simulink model "analyze"  (R2014a)
settings: Solver=FixedStepDiscrete  StartTime=0.0  StopTime=1  FixedStep=0.02  RelTol=1e-3
InitFcn:
  | Veh_Par_wxt
values from neighbouring files (symbols this model uses):
  ag_thr = 0.4*g    (= 3.924)    [Veh_Par_wxt.m]
  B = 2.25    [Veh_Par_wxt.m]
  bra_pre_em = 12    [Veh_Par_wxt.m]
  bra_pre_gz2 = 12/3    (= 4)    [Veh_Par_wxt.m]
  bra_pre_gz34 = 12/3    (= 4)    [Veh_Par_wxt.m]
  bra_pre_yd = 12/2    (= 6)    [Veh_Par_wxt.m]
  brakepre_dem_data = [0 1 2 3 4 5 6 7 8 9 10 11 12]    [Veh_Par_wxt.m]
  brakeTrq_dem_data = [0 218.198 436.396 654.594 872.792 1090.99 1309.188 1527.386 1745.584 1963.782 2181.98 2400.178 2618.376]    [Veh_Par_wxt.m]
  bratrq_max = 4*2618.376    (= 10473.504)    [Veh_Par_wxt.m]
  eff_tran = 0.75    [Veh_Par_wxt.m]
  G = Mass*g    (= 36297)    [Veh_Par_wxt.m]
  kd1 = 1    [Veh_Par_wxt.m]
  kd2 = 1    [Veh_Par_wxt.m]
  kd3 = 1    [Veh_Par_wxt.m]
  ki1 = 1    [Veh_Par_wxt.m]
  ki2 = 1    [Veh_Par_wxt.m]
  ki3 = 1    [Veh_Par_wxt.m]
  kp1 = 1    [Veh_Par_wxt.m]
  kp2 = 1    [Veh_Par_wxt.m]
  kp3 = 1    [Veh_Par_wxt.m]
  L = 3.12    [Veh_Par_wxt.m]
  premax = 12    [Veh_Par_wxt.m]
  Radius = 0.20    (= 0.2)    [Veh_Par_wxt.m]
  s_opt_yi_add = 0.05    [Veh_Par_wxt.m]
  s_opt_zhuan_add = 0.05    [Veh_Par_wxt.m]
  spd_map_mot = [0 100 200 300 360 400 500 600 700 800 900]*tras_ratio    [Veh_Par_wxt.m]
  spdmax = 900*tras_ratio    (= 5580)    [Veh_Par_wxt.m]
  speed_thr_park = 5/3.6/Radius*30/pi    (= 66.3145596216)    [Veh_Par_wxt.m]
  tras_ratio = 6.2    [Veh_Par_wxt.m]
  trq_map_mot = [1200 1200 1200 1200 1200 1080 864 720 617 540 480]/tras_ratio    [Veh_Par_wxt.m]
  trqmax = 80    [Veh_Par_wxt.m]
  v_thr1_b = 5    [Veh_Par_wxt.m]
  v_thr2_b = 20    [Veh_Par_wxt.m]
  v_thr_park = 5    [Veh_Par_wxt.m]
undefined symbols (not defined in the file or in its folder): DiscIntNeverNeededParam
libraries: simulink x231, ec5744lib x19
(part 13 of 16)

== system analyze/MainControl/mode_control/forward/forward/Drive/驱动防滑控制TCS ==
  trq_dem_lf : Inport
  trq_dem_lr : Inport  Port=2
  trq_dem_rf : Inport  Port=3
  trq_dem_rr : Inport  Port=4
  bra_pre_l : Inport  Port=5
  bra_pre_r : Inport  Port=6
  speed_act_lf : Inport  Port=7
  speed_act_lr : Inport  Port=8
  speed_act_rf : Inport  Port=9
  speed_act_rr : Inport  Port=10
  v_act : Inport  Port=11
  steer_dem : Inport  Port=12
  acc_y : Inport  Port=13
  brake_dem : Inport  Port=14
  s_opt_zhuan : Inport  Port=15
  MATLAB Function : MATLAB Function  TreatAsAtomicUnit=on
  Multiport Switch : MultiPortSwitch  DataPortOrder=Zero-based contiguous  Inputs=2
  Switch Case : SwitchCase  CaseConditions={0,1}  ShowDefaultCase=off
  直行TCS : Subsystem  TreatAsAtomicUnit=on
  转向TCS : Subsystem  TreatAsAtomicUnit=on
  forward_dem : Outport
  wires:
  steer_dem/1 -> 转向TCS/1(steer_dem), 直行TCS/1(steer_dem), MATLAB Function/1(steer_dem)
  MATLAB Function/1(y) -> Multiport Switch/1, Switch Case/1
  Switch Case/1 -> 转向TCS/Action
  Switch Case/2 -> 直行TCS/Action
  trq_dem_lf/1 -> 直行TCS/2(trq_dem_lf), 转向TCS/2(trq_dem_lf)
  trq_dem_lr/1 -> 直行TCS/3(trq_dem_lr), 转向TCS/3(trq_dem_lr)
  trq_dem_rf/1 -> 直行TCS/4(trq_dem_rf), 转向TCS/4(trq_dem_rf)
  trq_dem_rr/1 -> 直行TCS/5(trq_dem_rr), 转向TCS/5(trq_dem_rr)
  bra_pre_l/1 -> 直行TCS/6(bra_pre_l), 转向TCS/6(bra_pre_l)
  bra_pre_r/1 -> 直行TCS/7(bra_pre_r), 转向TCS/7(bra_pre_r)
  speed_act_lf/1 -> 直行TCS/8(speed_act_lf), 转向TCS/8(speed_act_lf)
  speed_act_lr/1 -> 直行TCS/9(speed_act_lr), 转向TCS/9(speed_act_lr)
  speed_act_rf/1 -> 直行TCS/10(speed_act_rf), 转向TCS/10(speed_act_rf)
  speed_act_rr/1 -> 直行TCS/11(speed_act_rr), 转向TCS/11(speed_act_rr)
  v_act/1 -> 直行TCS/12(v_act), 转向TCS/12(v_act)
  acc_y/1 -> 直行TCS/13(acc_y), 转向TCS/13(acc_y)
  s_opt_zhuan/1 -> 直行TCS/15(s_opt_zhuan), 转向TCS/15(s_opt_zhuan)
  brake_dem/1 -> 直行TCS/14(brake_dem), 转向TCS/14(brake_dem)
  直行TCS/1(forward_dem) -> Multiport Switch/3
  转向TCS/1(forward_dem) -> Multiport Switch/2
  Multiport Switch/1 -> forward_dem/1

== matlab function analyze/MainControl/mode_control/emergency_stop/emergency_stop/HeartBeat ==
  data: life_pre input; life output
function life = fcn(life_pre)
%#codegen
life=life_pre+1;
if life>15
    life=0;
end
end

== matlab function analyze/MainControl/mode_control/forward/forward/Drive/驱动防滑控制TCS/直行TCS/直行/MATLAB Function4 ==
  data: trq_dem_lf input; trq_dem_lr input; trq_dem_rf input; trq_dem_rr input; bra_pre_l input; bra_pre_r input; brakepre_dem input; flag_lf input; flag_lr input; trq_out_lf output; flag_rf input; flag_rr input; trq_out_lr output; trq_out_rf output; trq_out_rr output; trq_pid_lf input; trq_pid_lr input; trq_pid_rf input; trq_pid_rr input; brapre_out_l output; brapre_out_r output; mode output
function [trq_out_lf,trq_out_lr,trq_out_rf,trq_out_rr,brapre_out_l,brapre_out_r,mode] = fcn(trq_dem_lf,trq_dem_lr,trq_dem_rf,trq_dem_rr,bra_pre_l,bra_pre_r,brakepre_dem,flag_lf,flag_lr,flag_rf,flag_rr,trq_pid_lf,trq_pid_lr,trq_pid_rf,trq_pid_rr)
%#codegen pid模块在外面做，里面进行十六种情况的判断，先看一下效果，不能再修改。
if flag_lf==0 && flag_lr==0 && flag_rf==0 && flag_rr==0 % 0电机滑转===============================================0电机滑转
    trq_out_lf=trq_dem_lf;
    trq_out_lr=trq_dem_lr;
    trq_out_rf=trq_dem_rf;
    trq_out_rr=trq_dem_rr;
    brapre_out_l=bra_pre_l+brakepre_dem;
    brapre_out_r=bra_pre_r+brakepre_dem;
    mode=1;
elseif flag_lf==1 && flag_lr==0 &&flag_rf==0 && flag_rr==0 %左前轮滑转===================================================1电机滑转
    trq_out_lf=trq_pid_lf;
    trq_out_lr=trq_dem_lr+(trq_dem_lf-trq_out_lf);
    trq_out_rf=trq_dem_rf;
    trq_out_rr=trq_dem_rr;
    brapre_out_l=bra_pre_l+brakepre_dem;
    brapre_out_r=bra_pre_r+brakepre_dem;
    mode=2;
elseif flag_lf==0 && flag_lr==1 &&flag_rf==0 && flag_rr==0 %左后轮滑转
    trq_out_lr=trq_pid_lr;
    trq_out_lf=trq_dem_lf+(trq_dem_lr-trq_out_lr);
    trq_out_rf=trq_dem_rf;
    trq_out_rr=trq_dem_rr;
    brapre_out_l=bra_pre_l+brakepre_dem;
    brapre_out_r=bra_pre_r+brakepre_dem;
    mode=3;
elseif flag_lf==0 && flag_lr==0 &&flag_rf==1 && flag_rr==0 %右前轮滑转
    trq_out_rf=trq_pid_rf;
    trq_out_rr=trq_dem_rr+(trq_dem_rf-trq_out_rf);
    trq_out_lf=trq_dem_lf;
    trq_out_lr=trq_dem_lr;
    brapre_out_l=bra_pre_l+brakepre_dem;
    brapre_out_r=bra_pre_r+brakepre_dem;
    mode=4;
elseif flag_lf==0 && flag_lr==0 &&flag_rf==0 && flag_rr==1 %右后轮滑转
    trq_out_rr=trq_pid_rr;
    trq_out_rf=trq_dem_rf+(trq_dem_rr-trq_out_rr);
    trq_out_lf=trq_dem_lf;
    trq_out_lr=trq_dem_lr;
    brapre_out_l=bra_pre_l+brakepre_dem;
    brapre_out_r=bra_pre_r+brakepre_dem;
    mode=5;
elseif flag_lf==1 && flag_lr==1 &&flag_rf==0 && flag_rr==0 %左侧两轮滑转=====================================================================2电机滑转
    trq_out_lf=trq_pid_lf;
    trq_out_lr=trq_pid_lr;
    trq_out_rf=trq_dem_rf-(trq_dem_lf+trq_dem_lr-trq_out_lf-trq_out_lr)/2;
    trq_out_rr=trq_dem_rr-(trq_dem_lf+trq_dem_lr-trq_out_lf-trq_out_lr)/2;
    brapre_out_l=bra_pre_l+brakepre_dem;
    brapre_out_r=bra_pre_r+brakepre_dem;
    mode=6;
elseif flag_lf==0 && flag_lr==0 &&flag_rf==1 && flag_rr==1 %右侧两轮滑转
    trq_out_rf=trq_pid_rf;
    trq_out_rr=trq_pid_rr;
    trq_out_lf=trq_dem_lf-(trq_dem_rf+trq_dem_rr-trq_out_rf-trq_out_rr)/2;
    trq_out_lr=trq_dem_lr-(trq_dem_rf+trq_dem_rr-trq_out_rf-trq_out_rr)/2;
    brapre_out_l=bra_pre_l+brakepre_dem;
    brapre_out_r=bra_pre_r+brakepre_dem;
    mode=7;
elseif flag_lf==1 && flag_lr==0 &&flag_rf==1 && flag_rr==0 %前轴滑转
    trq_out_lf=trq_pid_lf;
    trq_out_lr=trq_dem_lr+(trq_dem_lf-trq_out_lf);
    trq_out_rf=trq_pid_rf;
    trq_out_rr=trq_dem_rr+(trq_dem_rf-trq_out_rf);
    brapre_out_l=bra_pre_l+brakepre_dem;
    brapre_out_r=bra_pre_r+brakepre_dem;
    mode=8;
elseif flag_lf==0 && flag_lr==1 &&flag_rf==0 && flag_rr==1 %后轴滑转
    trq_out_lr=trq_pid_lr;
    trq_out_lf=trq_dem_lf+(trq_dem_lr-trq_out_lr);
    trq_out_rr=trq_pid_rr;
    trq_out_rf=trq_dem_rf+(trq_dem_rr-trq_out_rr);
    brapre_out_l=bra_pre_l+brakepre_dem;
    brapre_out_r=bra_pre_r+brakepre_dem;
    mode=9;
elseif flag_lf==1 && flag_lr==0 &&flag_rf==0 && flag_rr==1 %左前轮和右后轮滑转
    trq_out_lf=trq_pid_lf;
    trq_out_lr=trq_dem_lr+(trq_dem_lf-trq_out_lf);
    trq_out_rr=trq_pid_rr;
    trq_out_rf=trq_dem_rf+(trq_dem_rr-trq_out_rr);
    brapre_out_l=bra_pre_l+brakepre_dem;
    brapre_out_r=bra_pre_r+brakepre_dem;
    mode=10;
elseif flag_lf==0 && flag_lr==1 &&flag_rf==1 && flag_rr==0 %左后轮和右前轮滑转
    trq_out_lr=trq_pid_lr;
    trq_out_lf=trq_dem_lf+(trq_dem_lr-trq_out_lr);
    trq_out_rf=trq_pid_rf;
    trq_out_rr=trq_dem_rr+(trq_dem_rf-trq_out_rf);
    brapre_out_l=bra_pre_l+brakepre_dem;
    brapre_out_r=bra_pre_r+brakepre_dem;
    mode=11;
elseif flag_lf==1 && flag_lr==1 &&flag_rf==1 && flag_rr==0 %右后不滑转======================================================================3电机滑转
    trq_out_lf=trq_pid_lf;
    trq_out_lr=trq_pid_lr;
    trq_out_rf=trq_pid_rf;
    trq_out_rr=trq_dem_rr+(trq_dem_rf-trq_out_rf)-(trq_dem_lf+trq_dem_lr-trq_out_lf-trq_out_lr);
    brapre_out_l=bra_pre_l+brakepre_dem;
    brapre_out_r=bra_pre_r+brakepre_dem;
    mode=12;
elseif flag_lf==1 && flag_lr==1 &&flag_rf==0 && flag_rr==1 %右前不滑转
    trq_out_lf=trq_pid_lf;
    trq_out_lr=trq_pid_lr;
    trq_out_rr=trq_pid_rr;
    trq_out_rf=trq_dem_rf+(trq_dem_rr-trq_out_rr)-(trq_dem_lf+trq_dem_lr-trq_out_lf-trq_out_lr);
    brapre_out_l=bra_pre_l+brakepre_dem;
    brapre_out_r=bra_pre_r+brakepre_dem;
    mode=13;
elseif flag_lf==1 && flag_lr==0 &&flag_rf==1 && flag_rr==1 %左后不滑转
    trq_out_rf=trq_pid_rf;
    trq_out_rr=trq_pid_rr;
    trq_out_lf=trq_pid_lf;
    trq_out_lr=trq_dem_lr+(trq_dem_lf-trq_out_lf)-(trq_dem_rf+trq_dem_rr-trq_out_rf-trq_out_rr);
    brapre_out_l=bra_pre_l+brakepre_dem;
    brapre_out_r=bra_pre_r+brakepre_dem;
    mode=14;
elseif flag_lf==0 && flag_lr==1 &&flag_rf==1 && flag_rr==1 %左前不滑转
    trq_out_rf=trq_pid_rf;
    trq_out_rr=trq_pid_rr;
    trq_out_lr=trq_pid_lr;
    trq_out_lf=trq_dem_lf+(trq_dem_lr-trq_out_lr)-(trq_dem_rf+trq_dem_rr-trq_out_rf-trq_out_rr);
    brapre_out_l=bra_pre_l+brakepre_dem;
    brapre_out_r=bra_pre_r+brakepre_dem;
    mode=15;
else
    %     flag_lf==1 && flag_lr==1 &&flag_rf==1 && flag_rr==1 %4电机均滑转======================================================================4电机均滑转
    trqcha=(trq_pid_lf+trq_pid_lr)-(trq_pid_rf+trq_pid_rr);
    if trqcha>0
        trq_out_rf=trq_pid_rf;
        trq_out_rr=trq_pid_rr;
        trq_out_lf=trq_pid_lf-(trq_pid_lf/(trq_pid_lf+trq_pid_lr))*trqcha;
        trq_out_lr=trq_pid_lr-(trq_pid_lr/(trq_pid_lf+trq_pid_lr))*trqcha;
    else
        trq_out_lf=trq_pid_lf;
        trq_out_lr=trq_pid_lr;
        trq_out_rf=trq_pid_rf+(trq_pid_rf/(trq_pid_rf+trq_pid_rr))*trqcha;
        trq_out_rr=trq_pid_rr+(trq_pid_rr/(trq_pid_rf+trq_pid_rr))*trqcha;
    end
    brapre_out_l=bra_pre_l+brakepre_dem;
    brapre_out_r=bra_pre_r+brakepre_dem;
    mode=16;
end
trq_out_lf=max(0,trq_out_lf);
trq_out_lr=max(0,trq_out_lr);
trq_out_rf=max(0,trq_out_rf);
trq_out_rr=max(0,trq_out_rr);
brapre_out_l=brapre_out_l;
brapre_out_r=brapre_out_r;
end

== system analyze/MainControl/mode_control/backward/backward/Drive/驱动防滑控制TCS/直行TCS ==
  steer_dem : Inport
  trq_dem_lf : Inport  Port=2
  trq_dem_lr : Inport  Port=3
  trq_dem_rf : Inport  Port=4
  trq_dem_rr : Inport  Port=5
  bra_pre_l : Inport  Port=6
  bra_pre_r : Inport  Port=7
  speed_act_lf : Inport  Port=8
  speed_act_lr : Inport  Port=9
  speed_act_rf : Inport  Port=10
  speed_act_rr : Inport  Port=11
  v_act : Inport  Port=12
  acc_y : Inport  Port=13
  brake_dem : Inport  Port=14
  s_opt_zhuan : Inport  Port=15
  Action Port : ActionPort  ActionType=case
  Scope : Scope  NumInputPorts=4
      settings: YMin=-5~-5~-5~-5  YMax=5~5~5~5  SaveName=ScopeData42
  Subsystem : Subsystem
  Subsystem1 : Subsystem
  Subsystem2 : Subsystem
  Subsystem3 : Subsystem
  Terminator : Terminator
  Terminator1 : Terminator
  直行 : Subsystem  TreatAsAtomicUnit=on
  backward_dem : Outport
  wires:
  steer_dem/1 -> Terminator1/1
  speed_act_lf/1 -> Subsystem/1(speed_act_lf)
  v_act/1 -> Subsystem2/2(v_act), Subsystem1/2(v_act), Subsystem/2(v_act), Subsystem3/2(v_act)
  speed_act_lr/1 -> Subsystem1/1(speed_act_lr)
  speed_act_rf/1 -> Subsystem2/1(speed_act_rf)
  speed_act_rr/1 -> Subsystem3/1(speed_act_rr)
  acc_y/1 -> Terminator/1
  trq_dem_lr/1 -> 直行/2(trq_dem_lr)
  trq_dem_lf/1 -> 直行/1(trq_dem_lf)
  trq_dem_rf/1 -> 直行/3(trq_dem_rf)
  trq_dem_rr/1 -> 直行/4(trq_dem_rr)
  bra_pre_l/1 -> 直行/5(bra_pre_l)
  bra_pre_r/1 -> 直行/6(bra_pre_r)
  Subsystem/1(s_act_lf) -> 直行/7(s_act_lf), Scope/1
  Subsystem1/1(s_act_lr) -> 直行/8(s_act_lr), Scope/2
  Subsystem2/1(s_act_rf) -> 直行/9(s_act_rf), Scope/3
  Subsystem3/1(s_act_rr) -> 直行/10(s_act_rr), Scope/4
  s_opt_zhuan/1 -> 直行/12(s_opt_zhuan)
  brake_dem/1 -> 直行/11(brake_dem)
  直行/1(backward_dem) -> backward_dem/1

== system analyze/MainControl/mode_control/backward/backward/Drive/驱动防滑控制TCS/转向TCS ==
  steer_dem : Inport
  trq_dem_lf : Inport  Port=2
  trq_dem_lr : Inport  Port=3
  trq_dem_rf : Inport  Port=4
  trq_dem_rr : Inport  Port=5
  bra_pre_l : Inport  Port=6
  bra_pre_r : Inport  Port=7
  speed_act_lf : Inport  Port=8
  speed_act_lr : Inport  Port=9
  speed_act_rf : Inport  Port=10
  speed_act_rr : Inport  Port=11
  v_act : Inport  Port=12
  acc_y : Inport  Port=13
  brake_dem : Inport  Port=14
  s_opt_zhuan : Inport  Port=15
  Action Port : ActionPort  ActionType=case
  MATLAB Function : MATLAB Function  TreatAsAtomicUnit=on
  Multiport Switch : MultiPortSwitch  DataPortOrder=Zero-based contiguous  Inputs=2
  Subsystem : Subsystem
  Subsystem1 : Subsystem
  Subsystem2 : Subsystem
  Subsystem3 : Subsystem
  Switch Case : SwitchCase  CaseConditions={0,1}  ShowDefaultCase=off
  Terminator : Terminator
  右转 : Subsystem  TreatAsAtomicUnit=on
  左转 : Subsystem  TreatAsAtomicUnit=on
  backward_dem : Outport
  wires:
  Multiport Switch/1 -> backward_dem/1
  右转/1(backward_dem) -> Multiport Switch/3
  左转/1(backward_dem) -> Multiport Switch/2
  brake_dem/1 -> 左转/11(brake_dem), 右转/11(brake_dem)
  s_opt_zhuan/1 -> 左转/12(s_opt_zhuan), 右转/12(s_opt_zhuan)
  Subsystem3/1(s_act_rr) -> 左转/10(s_act_rr), 右转/10(s_act_rr)
  Subsystem2/1(s_act_rf) -> 左转/9(s_act_rf), 右转/9(s_act_rf)
  Subsystem1/1(s_act_lr) -> 左转/8(s_act_lr), 右转/8(s_act_lr)
  Subsystem/1(s_act_lf) -> 左转/7(s_act_lf), 右转/7(s_act_lf)
  bra_pre_r/1 -> 左转/6(bra_pre_r), 右转/6(bra_pre_r)
  bra_pre_l/1 -> 左转/5(bra_pre_l), 右转/5(bra_pre_l)
  trq_dem_rr/1 -> 左转/4(trq_dem_rr), 右转/4(trq_dem_rr)
  trq_dem_rf/1 -> 左转/3(trq_dem_rf), 右转/3(trq_dem_rf)
  trq_dem_lf/1 -> 左转/1(trq_dem_lf), 右转/1(trq_dem_lf)
  trq_dem_lr/1 -> 左转/2(trq_dem_lr), 右转/2(trq_dem_lr)
  acc_y/1 -> Terminator/1
  Switch Case/2 -> 右转/Action
  Switch Case/1 -> 左转/Action
  speed_act_rr/1 -> Subsystem3/1(speed_act_rr)
  speed_act_rf/1 -> Subsystem2/1(speed_act_rf)
  speed_act_lr/1 -> Subsystem1/1(speed_act_lr)
  v_act/1 -> Subsystem3/2(v_act), Subsystem/2(v_act), Subsystem1/2(v_act), Subsystem2/2(v_act)
  speed_act_lf/1 -> Subsystem/1(speed_act_lf)
  MATLAB Function/1(y) -> Switch Case/1, Multiport Switch/1
  steer_dem/1 -> MATLAB Function/1(steer_dem)

== system analyze/MainControl/mode_control/forward/forward/Drive/驱动防滑控制TCS/直行TCS ==
  steer_dem : Inport
  trq_dem_lf : Inport  Port=2
  trq_dem_lr : Inport  Port=3
  trq_dem_rf : Inport  Port=4
  trq_dem_rr : Inport  Port=5
  bra_pre_l : Inport  Port=6
  bra_pre_r : Inport  Port=7
  speed_act_lf : Inport  Port=8
  speed_act_lr : Inport  Port=9
  speed_act_rf : Inport  Port=10
  speed_act_rr : Inport  Port=11
  v_act : Inport  Port=12
  acc_y : Inport  Port=13
  brake_dem : Inport  Port=14
  s_opt_zhuan : Inport  Port=15
  Action Port : ActionPort  ActionType=case
  Scope : Scope  NumInputPorts=4
      settings: YMin=-5~-5~-5~-5  YMax=5~5~5~5  SaveName=ScopeData42
  Subsystem : Subsystem
  Subsystem1 : Subsystem
  Subsystem2 : Subsystem
  Subsystem3 : Subsystem
  Terminator : Terminator
  Terminator1 : Terminator
  直行 : Subsystem  TreatAsAtomicUnit=on
  forward_dem : Outport
  wires:
  直行/1(forward_dem) -> forward_dem/1
  brake_dem/1 -> 直行/11(brake_dem)
  s_opt_zhuan/1 -> 直行/12(s_opt_zhuan)
  Subsystem3/1(s_act_rr) -> Scope/4, 直行/10(s_act_rr)
  Subsystem2/1(s_act_rf) -> Scope/3, 直行/9(s_act_rf)
  Subsystem1/1(s_act_lr) -> Scope/2, 直行/8(s_act_lr)
  Subsystem/1(s_act_lf) -> Scope/1, 直行/7(s_act_lf)
  bra_pre_r/1 -> 直行/6(bra_pre_r)
  bra_pre_l/1 -> 直行/5(bra_pre_l)
  trq_dem_rr/1 -> 直行/4(trq_dem_rr)
  trq_dem_rf/1 -> 直行/3(trq_dem_rf)
  trq_dem_lf/1 -> 直行/1(trq_dem_lf)
  trq_dem_lr/1 -> 直行/2(trq_dem_lr)
  acc_y/1 -> Terminator/1
  speed_act_rr/1 -> Subsystem3/1(speed_act_rr)
  speed_act_rf/1 -> Subsystem2/1(speed_act_rf)
  speed_act_lr/1 -> Subsystem1/1(speed_act_lr)
  v_act/1 -> Subsystem3/2(v_act), Subsystem/2(v_act), Subsystem1/2(v_act), Subsystem2/2(v_act)
  speed_act_lf/1 -> Subsystem/1(speed_act_lf)
  steer_dem/1 -> Terminator1/1

== system analyze/MainControl/mode_control/forward/forward/Drive/驱动防滑控制TCS/转向TCS ==
  steer_dem : Inport
  trq_dem_lf : Inport  Port=2
  trq_dem_lr : Inport  Port=3
  trq_dem_rf : Inport  Port=4
  trq_dem_rr : Inport  Port=5
  bra_pre_l : Inport  Port=6
  bra_pre_r : Inport  Port=7
  speed_act_lf : Inport  Port=8
  speed_act_lr : Inport  Port=9
  speed_act_rf : Inport  Port=10
  speed_act_rr : Inport  Port=11
  v_act : Inport  Port=12
  acc_y : Inport  Port=13
  brake_dem : Inport  Port=14
  s_opt_zhuan : Inport  Port=15
  Action Port : ActionPort  ActionType=case
  MATLAB Function : MATLAB Function  TreatAsAtomicUnit=on
  Multiport Switch : MultiPortSwitch  DataPortOrder=Zero-based contiguous  Inputs=2
  Subsystem : Subsystem
  Subsystem1 : Subsystem
  Subsystem2 : Subsystem
  Subsystem3 : Subsystem
  Switch Case : SwitchCase  CaseConditions={0,1}  ShowDefaultCase=off
  Terminator : Terminator
  右转 : Subsystem  TreatAsAtomicUnit=on
  左转 : Subsystem  TreatAsAtomicUnit=on
  forward_dem : Outport
  wires:
  steer_dem/1 -> MATLAB Function/1(steer_dem)
  MATLAB Function/1(y) -> Multiport Switch/1, Switch Case/1
  speed_act_lf/1 -> Subsystem/1(speed_act_lf)
  v_act/1 -> Subsystem2/2(v_act), Subsystem1/2(v_act), Subsystem/2(v_act), Subsystem3/2(v_act)
  speed_act_lr/1 -> Subsystem1/1(speed_act_lr)
  speed_act_rf/1 -> Subsystem2/1(speed_act_rf)
  speed_act_rr/1 -> Subsystem3/1(speed_act_rr)
  Switch Case/1 -> 左转/Action
  Switch Case/2 -> 右转/Action
  acc_y/1 -> Terminator/1
  trq_dem_lr/1 -> 右转/2(trq_dem_lr), 左转/2(trq_dem_lr)
  trq_dem_lf/1 -> 右转/1(trq_dem_lf), 左转/1(trq_dem_lf)
  trq_dem_rf/1 -> 右转/3(trq_dem_rf), 左转/3(trq_dem_rf)
  trq_dem_rr/1 -> 右转/4(trq_dem_rr), 左转/4(trq_dem_rr)
  bra_pre_l/1 -> 右转/5(bra_pre_l), 左转/5(bra_pre_l)
  bra_pre_r/1 -> 右转/6(bra_pre_r), 左转/6(bra_pre_r)
  Subsystem/1(s_act_lf) -> 右转/7(s_act_lf), 左转/7(s_act_lf)
  Subsystem1/1(s_act_lr) -> 右转/8(s_act_lr), 左转/8(s_act_lr)
  Subsystem2/1(s_act_rf) -> 右转/9(s_act_rf), 左转/9(s_act_rf)
  Subsystem3/1(s_act_rr) -> 右转/10(s_act_rr), 左转/10(s_act_rr)
  s_opt_zhuan/1 -> 右转/12(s_opt_zhuan), 左转/12(s_opt_zhuan)
  brake_dem/1 -> 右转/11(brake_dem), 左转/11(brake_dem)
  左转/1(forward_dem) -> Multiport Switch/2
  右转/1(forward_dem) -> Multiport Switch/3
  Multiport Switch/1 -> forward_dem/1

== system analyze/MainControl/mode_control/backward/backward/Drive/驱动防滑控制TCS/直行TCS/Subsystem ==
  speed_act_lf : Inport
  v_act : Inport  Port=2
  Add : Sum
  Constant : Constant  Value=eps
  Divide : Product  Inputs=*/
  Gain : Gain  Gain=pi/30
  Gain1 : Gain  Gain=Radius
  Gain2 : Gain  Gain=1/3.6
  Subtract : Sum  Inputs=+-
  s_act_lf : Outport
  wires:
  speed_act_lf/1 -> Gain/1
  Gain/1 -> Gain1/1
  v_act/1 -> Gain2/1
  Gain1/1 -> Add/1, Subtract/1
  Gain2/1 -> Subtract/2
  Subtract/1 -> Divide/1
  Constant/1 -> Add/2
  Add/1 -> Divide/2
  Divide/1 -> s_act_lf/1

== system analyze/MainControl/mode_control/backward/backward/Drive/驱动防滑控制TCS/直行TCS/Subsystem1 ==
  speed_act_lr : Inport
  v_act : Inport  Port=2
  Add : Sum
  Constant : Constant  Value=eps
  Divide : Product  Inputs=*/
  Gain : Gain  Gain=pi/30
  Gain1 : Gain  Gain=Radius
  Gain2 : Gain  Gain=1/3.6
  Subtract : Sum  Inputs=+-
  s_act_lr : Outport
  wires:
  Divide/1 -> s_act_lr/1
  Add/1 -> Divide/2
  Constant/1 -> Add/2
  Subtract/1 -> Divide/1
  Gain2/1 -> Subtract/2
  Gain1/1 -> Subtract/1, Add/1
  v_act/1 -> Gain2/1
  Gain/1 -> Gain1/1
  speed_act_lr/1 -> Gain/1

== system analyze/MainControl/mode_control/backward/backward/Drive/驱动防滑控制TCS/直行TCS/Subsystem2 ==
  speed_act_rf : Inport
  v_act : Inport  Port=2
  Add : Sum
  Constant : Constant  Value=eps
  Divide : Product  Inputs=*/
  Gain : Gain  Gain=pi/30
  Gain1 : Gain  Gain=Radius
  Gain2 : Gain  Gain=1/3.6
  Subtract : Sum  Inputs=+-
  s_act_rf : Outport
  wires:
  speed_act_rf/1 -> Gain/1
  Gain/1 -> Gain1/1
  v_act/1 -> Gain2/1
  Gain1/1 -> Add/1, Subtract/1
  Gain2/1 -> Subtract/2
  Subtract/1 -> Divide/1
  Constant/1 -> Add/2
  Add/1 -> Divide/2
  Divide/1 -> s_act_rf/1

== system analyze/MainControl/mode_control/backward/backward/Drive/驱动防滑控制TCS/直行TCS/Subsystem3 ==
  speed_act_rr : Inport
  v_act : Inport  Port=2
  Add : Sum
  Constant : Constant  Value=eps
  Divide : Product  Inputs=*/
  Gain : Gain  Gain=pi/30
  Gain1 : Gain  Gain=Radius
  Gain2 : Gain  Gain=1/3.6
  Subtract : Sum  Inputs=+-
  s_act_rr : Outport
  wires:
  Divide/1 -> s_act_rr/1
  Add/1 -> Divide/2
  Constant/1 -> Add/2
  Subtract/1 -> Divide/1
  Gain2/1 -> Subtract/2
  Gain1/1 -> Subtract/1, Add/1
  v_act/1 -> Gain2/1
  Gain/1 -> Gain1/1
  speed_act_rr/1 -> Gain/1

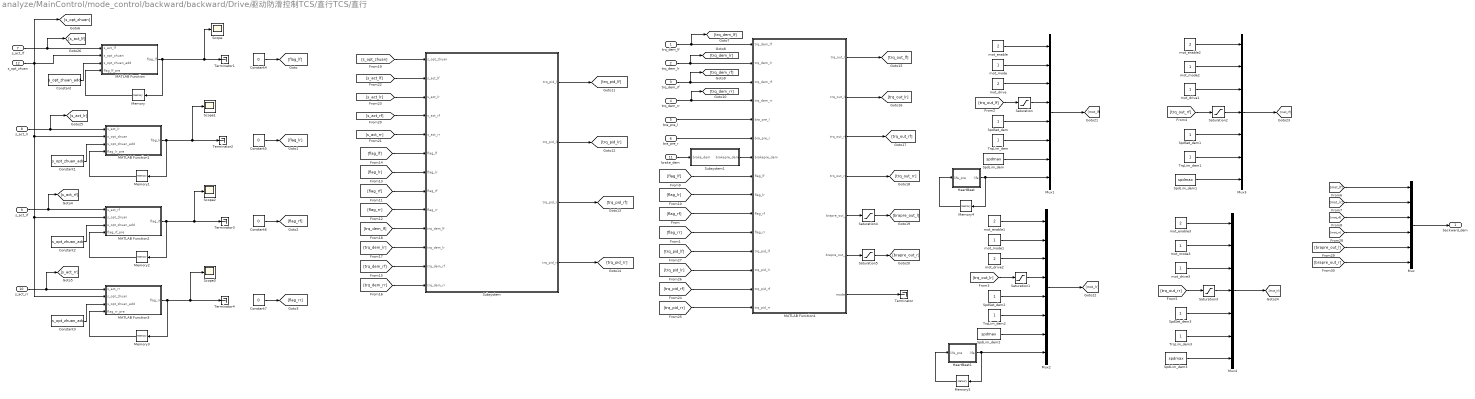
== system analyze/MainControl/mode_control/backward/backward/Drive/驱动防滑控制TCS/直行TCS/直行 ==
  trq_dem_lf : Inport
  trq_dem_lr : Inport  Port=2
  trq_dem_rf : Inport  Port=3
  trq_dem_rr : Inport  Port=4
  bra_pre_l : Inport  Port=5
  bra_pre_r : Inport  Port=6
  s_act_lf : Inport  Port=7
  s_act_lr : Inport  Port=8
  s_act_rf : Inport  Port=9
  s_act_rr : Inport  Port=10
  brake_dem : Inport  Port=11
  s_opt_zhuan : Inport  Port=12
  Constant{,1..3} (4 alike) : Constant  Value=s_opt_zhuan_add
  Constant{4..7} (4 alike) : Constant  Value=0
  HeartBeat : MATLAB Function  TreatAsAtomicUnit=on
  HeartBeat1 : MATLAB Function  TreatAsAtomicUnit=on
  MATLAB Function : MATLAB Function  TreatAsAtomicUnit=on
  MATLAB Function1 : MATLAB Function  TreatAsAtomicUnit=on
  MATLAB Function2 : MATLAB Function  TreatAsAtomicUnit=on
  MATLAB Function3 : MATLAB Function  TreatAsAtomicUnit=on
  MATLAB Function4 : MATLAB Function  TreatAsAtomicUnit=on
  Memory{,1..5} (6 alike) : Memory  InheritSampleTime=on
  Mux : Mux  Inputs=6
  Mux1 : Mux  Inputs=8
  Mux2 : Mux  Inputs=8
  Mux3 : Mux  Inputs=7
  Mux4 : Mux  Inputs=7
  Saturation{,1..3} (4 alike) : Saturate  UpperLimit=trqmax  LowerLimit=0
  Saturation4 : Saturate  UpperLimit=premax  LowerLimit=0
  Saturation5 : Saturate  UpperLimit=premax  LowerLimit=0
  Scope{,1..3} (4 alike) : Scope
      Scope settings: SaveName=ScopeData43
      Scope1 settings: SaveName=ScopeData44
      Scope2 settings: SaveName=ScopeData45
      Scope3 settings: SaveName=ScopeData46
  SpdLim_dem{,1..3} (4 alike) : Constant  Value=spdmax
  SpdSet_dem{,1..3} (4 alike) : Constant
  Subsystem : Subsystem
  Subsystem1 : Subsystem
  Terminator{,1..4} (5 alike) : Terminator
  TrqLim_dem{,1..3} (4 alike) : Constant
  mot_drive : Constant  Value=2
  mot_drive1 : Constant
  mot_drive2 : Constant  Value=2
  mot_drive3 : Constant
  mot_enable{,1..3} (4 alike) : Constant  Value=2
  mot_mode{,1..3} (4 alike) : Constant
  backward_dem : Outport
  wires:
  Saturation5/1 -> [brapre_out_r]
  Saturation4/1 -> [brapre_out_l]
  Saturation3/1 -> Mux4/4
  Saturation1/1 -> Mux2/4
  Saturation2/1 -> Mux3/4
  Saturation/1 -> Mux1/4
  MATLAB Function4/7(mode) -> Terminator/1
  brake_dem/1 -> Subsystem1/1(brake_dem)
  Subsystem1/1(brakepre_dem) -> MATLAB Function4/7(brakepre_dem)
  [brapre_out_r] -> Mux/6
  [brapre_out_l] -> Mux/5
  [mot_rr] -> Mux/4
  [mot_rf] -> Mux/3
  [mot_lr] -> Mux/2
  [mot_lf] -> Mux/1
  MATLAB Function4/6(brapre_out_r) -> Saturation5/1
  MATLAB Function4/5(brapre_out_l) -> Saturation4/1
  MATLAB Function4/4(trq_out_rr) -> [trq_out_rr]
  MATLAB Function4/3(trq_out_rf) -> [trq_out_rf]
  MATLAB Function4/2(trq_out_lr) -> [trq_out_lr]
  MATLAB Function4/1(trq_out_lf) -> [trq_out_lf]
  mot_drive/1 -> Mux1/3
  mot_mode/1 -> Mux1/2
  [trq_out_lf] -> Saturation/1
  mot_enable/1 -> Mux1/1
  SpdSet_dem/1 -> Mux1/5
  Mux1/1 -> [mot_lf]
  TrqLim_dem/1 -> Mux1/6
  HeartBeat/1(life) -> Mux1/8, Memory4/1
  Memory4/1 -> HeartBeat/1(life_pre)
  SpdLim_dem/1 -> Mux1/7
  mot_drive1/1 -> Mux3/3
  mot_mode2/1 -> Mux3/2
  [trq_out_rf] -> Saturation2/1
  mot_enable2/1 -> Mux3/1
  SpdSet_dem1/1 -> Mux3/5
  Mux3/1 -> [mot_rf]
  TrqLim_dem1/1 -> Mux3/6
  SpdLim_dem1/1 -> Mux3/7
  mot_drive2/1 -> Mux2/3
  mot_mode1/1 -> Mux2/2
  [trq_out_lr] -> Saturation1/1
  mot_enable1/1 -> Mux2/1
  SpdSet_dem2/1 -> Mux2/5
  Mux2/1 -> [mot_lr]
  TrqLim_dem2/1 -> Mux2/6
  HeartBeat1/1(life) -> Mux2/8, Memory5/1
  Memory5/1 -> HeartBeat1/1(life_pre)
  SpdLim_dem2/1 -> Mux2/7
  mot_drive3/1 -> Mux4/3
  mot_mode3/1 -> Mux4/2
  [trq_out_rr] -> Saturation3/1
  mot_enable3/1 -> Mux4/1
  SpdSet_dem3/1 -> Mux4/5
  Mux4/1 -> [mot_rr]
  TrqLim_dem3/1 -> Mux4/6
  SpdLim_dem3/1 -> Mux4/7
  bra_pre_r/1 -> MATLAB Function4/6(bra_pre_r)
  bra_pre_l/1 -> MATLAB Function4/5(bra_pre_l)
  trq_dem_rr/1 -> [trq_dem_rr], MATLAB Function4/4(trq_dem_rr)
  trq_dem_rf/1 -> [trq_dem_rf], MATLAB Function4/3(trq_dem_rf)
  trq_dem_lr/1 -> [trq_dem_lr], MATLAB Function4/2(trq_dem_lr)
  trq_dem_lf/1 -> [trq_dem_lf], MATLAB Function4/1(trq_dem_lf)
  [trq_pid_rr] -> MATLAB Function4/15(trq_pid_rr)
  [trq_pid_rf] -> MATLAB Function4/14(trq_pid_rf)
  [trq_pid_lr] -> MATLAB Function4/13(trq_pid_lr)
  [trq_pid_lf] -> MATLAB Function4/12(trq_pid_lf)
  Subsystem/3(trq_pid_rf) -> [trq_pid_rf]
  Subsystem/4(trq_pid_rr) -> [trq_pid_rr]
  Subsystem/1(trq_pid_lf) -> [trq_pid_lf]
  Subsystem/2(trq_pid_lr) -> [trq_pid_lr]
  [s_act_lf] -> Subsystem/2(s_act_lf)
  [s_act_lr] -> Subsystem/3(s_act_lr)
  [s_act_rf] -> Subsystem/4(s_act_rf)
  [s_act_rr] -> Subsystem/5(s_act_rr)
  [s_opt_zhuan] -> Subsystem/1(s_opt_zhuan)
  [flag_rr] -> Subsystem/9(flag_rr)
  [trq_dem_rr] -> Subsystem/13(trq_dem_rr)
  [flag_rf] -> Subsystem/8(flag_rf)
  [flag_lr] -> Subsystem/7(flag_lr)
  [trq_dem_lr] -> Subsystem/11(trq_dem_lr)
  [trq_dem_rf] -> Subsystem/12(trq_dem_rf)
  [flag_lf] -> Subsystem/6(flag_lf)
  [trq_dem_lf] -> Subsystem/10(trq_dem_lf)
  [flag_lf] -> MATLAB Function4/8(flag_lf)
  [flag_lr] -> MATLAB Function4/9(flag_lr)
  s_act_lf/1 -> MATLAB Function/1(s_act_lf), [s_act_lf]
  MATLAB Function/1(flag_lf) -> Memory/1, Terminator1/1, Scope/1
  Memory/1 -> MATLAB Function/4(flag_lf_pre)
  Constant/1 -> MATLAB Function/3(s_opt_zhuan_add)
  s_act_lr/1 -> MATLAB Function1/1(s_act_lr), [s_act_lr]
  MATLAB Function1/1(flag_lr) -> Terminator2/1, Scope1/1, Memory1/1
  Memory1/1 -> MATLAB Function1/4(flag_lr_pre)
  Constant1/1 -> MATLAB Function1/3(s_opt_zhuan_add)
  s_act_rf/1 -> [s_act_rf], MATLAB Function2/1(s_act_rf)
  MATLAB Function2/1(flag_rf) -> Memory2/1, Terminator3/1, Scope2/1
  Memory2/1 -> MATLAB Function2/4(flag_rf_pre)
  Constant2/1 -> MATLAB Function2/3(s_opt_zhuan_add)
  s_act_rr/1 -> [s_act_rr], MATLAB Function3/1(s_act_rr)
  s_opt_zhuan/1 -> [s_opt_zhuan], MATLAB Function3/2(s_opt_zhuan), MATLAB Function2/2(s_opt_zhuan), MATLAB Function1/2(s_opt_zhuan), MATLAB Function/2(s_opt_zhuan)
  MATLAB Function3/1(flag_rr) -> Terminator4/1, Scope3/1, Memory3/1
  Memory3/1 -> MATLAB Function3/4(flag_rr_pre)
  Constant3/1 -> MATLAB Function3/3(s_opt_zhuan_add)
  [flag_rf] -> MATLAB Function4/10(flag_rf)
  [flag_rr] -> MATLAB Function4/11(flag_rr)
  Mux/1 -> backward_dem/1
  Constant4/1 -> [flag_lf]
  Constant5/1 -> [flag_lr]
  Constant6/1 -> [flag_rf]
  Constant7/1 -> [flag_rr]

== system analyze/MainControl/mode_control/backward/backward/Drive/驱动防滑控制TCS/转向TCS/Subsystem ==
  speed_act_lf : Inport
  v_act : Inport  Port=2
  Add : Sum
  Constant : Constant  Value=eps
  Divide : Product  Inputs=*/
  Gain : Gain  Gain=pi/30
  Gain1 : Gain  Gain=Radius
  Gain2 : Gain  Gain=1/3.6
  Subtract : Sum  Inputs=+-
  s_act_lf : Outport
  wires:
  Divide/1 -> s_act_lf/1
  Add/1 -> Divide/2
  Constant/1 -> Add/2
  Subtract/1 -> Divide/1
  Gain2/1 -> Subtract/2
  Gain1/1 -> Subtract/1, Add/1
  v_act/1 -> Gain2/1
  Gain/1 -> Gain1/1
  speed_act_lf/1 -> Gain/1

== system analyze/MainControl/mode_control/backward/backward/Drive/驱动防滑控制TCS/转向TCS/Subsystem1 ==
  speed_act_lr : Inport
  v_act : Inport  Port=2
  Add : Sum
  Constant : Constant  Value=eps
  Divide : Product  Inputs=*/
  Gain : Gain  Gain=pi/30
  Gain1 : Gain  Gain=Radius
  Gain2 : Gain  Gain=1/3.6
  Subtract : Sum  Inputs=+-
  s_act_lr : Outport
  wires:
  speed_act_lr/1 -> Gain/1
  Gain/1 -> Gain1/1
  v_act/1 -> Gain2/1
  Gain1/1 -> Add/1, Subtract/1
  Gain2/1 -> Subtract/2
  Subtract/1 -> Divide/1
  Constant/1 -> Add/2
  Add/1 -> Divide/2
  Divide/1 -> s_act_lr/1

== system analyze/MainControl/mode_control/backward/backward/Drive/驱动防滑控制TCS/转向TCS/Subsystem2 ==
  speed_act_rf : Inport
  v_act : Inport  Port=2
  Add : Sum
  Constant : Constant  Value=eps
  Divide : Product  Inputs=*/
  Gain : Gain  Gain=pi/30
  Gain1 : Gain  Gain=Radius
  Gain2 : Gain  Gain=1/3.6
  Subtract : Sum  Inputs=+-
  s_act_rf : Outport
  wires:
  Divide/1 -> s_act_rf/1
  Add/1 -> Divide/2
  Constant/1 -> Add/2
  Subtract/1 -> Divide/1
  Gain2/1 -> Subtract/2
  Gain1/1 -> Subtract/1, Add/1
  v_act/1 -> Gain2/1
  Gain/1 -> Gain1/1
  speed_act_rf/1 -> Gain/1

== system analyze/MainControl/mode_control/backward/backward/Drive/驱动防滑控制TCS/转向TCS/Subsystem3 ==
  speed_act_rr : Inport
  v_act : Inport  Port=2
  Add : Sum
  Constant : Constant  Value=eps
  Divide : Product  Inputs=*/
  Gain : Gain  Gain=pi/30
  Gain1 : Gain  Gain=Radius
  Gain2 : Gain  Gain=1/3.6
  Subtract : Sum  Inputs=+-
  s_act_rr : Outport
  wires:
  speed_act_rr/1 -> Gain/1
  Gain/1 -> Gain1/1
  v_act/1 -> Gain2/1
  Gain1/1 -> Add/1, Subtract/1
  Gain2/1 -> Subtract/2
  Subtract/1 -> Divide/1
  Constant/1 -> Add/2
  Add/1 -> Divide/2
  Divide/1 -> s_act_rr/1

== system analyze/MainControl/mode_control/backward/backward/Drive/驱动防滑控制TCS/转向TCS/右转 ==
  trq_dem_lf : Inport
  trq_dem_lr : Inport  Port=2
  trq_dem_rf : Inport  Port=3
  trq_dem_rr : Inport  Port=4
  bra_pre_l : Inport  Port=5
  bra_pre_r : Inport  Port=6
  s_act_lf : Inport  Port=7
  s_act_lr : Inport  Port=8
  s_act_rf : Inport  Port=9
  s_act_rr : Inport  Port=10
  brake_dem : Inport  Port=11
  s_opt_zhuan : Inport  Port=12
  Action Port : ActionPort  ActionType=case
  Constant{,1..3} (4 alike) : Constant  Value=s_opt_zhuan_add
  Constant4 : Constant  Value=0
  Constant5 : Constant  Value=0
  MATLAB Function : MATLAB Function  TreatAsAtomicUnit=on
  MATLAB Function1 : MATLAB Function  TreatAsAtomicUnit=on
  MATLAB Function2 : MATLAB Function  TreatAsAtomicUnit=on
  MATLAB Function3 : MATLAB Function  TreatAsAtomicUnit=on
  MATLAB Function4 : MATLAB Function  TreatAsAtomicUnit=on
  Memory{,1..3} (4 alike) : Memory  InheritSampleTime=on
  Multiport Switch : MultiPortSwitch  DataPortOrder=Zero-based contiguous  Inputs=4
  Mux{,1..3} (4 alike) : Mux  Inputs=6
  Switch Case : SwitchCase  CaseConditions={0,1,2,3}  ShowDefaultCase=off
  Terminator{,1..3} (4 alike) : Terminator
  前后轮均滑转 : Subsystem  TreatAsAtomicUnit=on
  前轮滑转 : Subsystem  TreatAsAtomicUnit=on
  后轮滑转 : Subsystem  TreatAsAtomicUnit=on
  无滑转 : Subsystem  TreatAsAtomicUnit=on
  backward_dem : Outport
  wires:
  s_act_lf/1 -> MATLAB Function/1(s_act_lf), [s_act_lf]
  MATLAB Function/1(flag_lf) -> Terminator2/1, Memory/1
  Memory/1 -> MATLAB Function/4(flag_lf_pre)
  Constant/1 -> MATLAB Function/3(s_opt_zhuan_add)
  s_act_lr/1 -> MATLAB Function1/1(s_act_lr), [s_act_lr]
  MATLAB Function1/1(flag_lr) -> Terminator3/1, Memory1/1
  Memory1/1 -> MATLAB Function1/4(flag_lr_pre)
  Constant1/1 -> MATLAB Function1/3(s_opt_zhuan_add)
  s_act_rf/1 -> MATLAB Function2/1(s_act_rf)
  MATLAB Function2/1(flag_rf) -> Memory2/1, Terminator/1
  Memory2/1 -> MATLAB Function2/4(flag_rf_pre)
  Constant2/1 -> MATLAB Function2/3(s_opt_zhuan_add)
  s_act_rr/1 -> MATLAB Function3/1(s_act_rr)
  s_opt_zhuan/1 -> [s_opt_zhuan], MATLAB Function3/2(s_opt_zhuan), MATLAB Function2/2(s_opt_zhuan), MATLAB Function1/2(s_opt_zhuan), MATLAB Function/2(s_opt_zhuan)
  MATLAB Function3/1(flag_rr) -> Memory3/1, Terminator1/1
  Memory3/1 -> MATLAB Function3/4(flag_rr_pre)
  Constant3/1 -> MATLAB Function3/3(s_opt_zhuan_add)
  [flag_lf] -> MATLAB Function4/1(flag_lf)
  [flag_lr] -> MATLAB Function4/2(flag_lr)
  MATLAB Function4/1(y) -> Multiport Switch/1, Switch Case/1
  Switch Case/1 -> 无滑转/Action
  trq_dem_lf/1 -> 无滑转/1(trq_dem_lf), 前后轮均滑转/1(trq_dem_lf), 后轮滑转/1(trq_dem_lf), 前轮滑转/1(trq_dem_lf)
  trq_dem_lr/1 -> 无滑转/2(trq_dem_lr), 前轮滑转/2(trq_dem_lr), 前后轮均滑转/2(trq_dem_lr), 后轮滑转/2(trq_dem_lr)
  trq_dem_rf/1 -> 无滑转/3(trq_dem_rf), 前后轮均滑转/3(trq_dem_rf), 后轮滑转/3(trq_dem_rf), 前轮滑转/3(trq_dem_rf)
  trq_dem_rr/1 -> 无滑转/4(trq_dem_rr), 前后轮均滑转/4(trq_dem_rr), 后轮滑转/4(trq_dem_rr), 前轮滑转/4(trq_dem_rr)
  bra_pre_l/1 -> 无滑转/5(bra_pre_l), 前后轮均滑转/5(bra_pre_l), 后轮滑转/5(bra_pre_l), 前轮滑转/5(bra_pre_l)
  bra_pre_r/1 -> 无滑转/6(bra_pre_r), 前后轮均滑转/6(bra_pre_r), 后轮滑转/6(bra_pre_r), 前轮滑转/6(bra_pre_r)
  brake_dem/1 -> 无滑转/7(brake_dem), 前后轮均滑转/7(brake_dem), 后轮滑转/7(brake_dem), 前轮滑转/7(brake_dem)
  无滑转/1(mot_lf) -> Mux/1
  无滑转/2(mot_lr) -> Mux/2
  无滑转/4(mot_rr) -> Mux/4
  无滑转/3(mot_rf) -> Mux/3
  无滑转/5(bra_pre_l1) -> Mux/5
  无滑转/6(bra_pre_r1) -> Mux/6
  Mux/1 -> Multiport Switch/2
  Multiport Switch/1 -> backward_dem/1
  Switch Case/2 -> 前轮滑转/Action
  前轮滑转/6(bra_pre_r1) -> Mux1/6
  前轮滑转/3(mot_rf) -> Mux1/3
  前轮滑转/2(mot_lr) -> Mux1/2
  前轮滑转/1(mot_lf) -> Mux1/1
  前轮滑转/5(bra_pre_l1) -> Mux1/5
  前轮滑转/4(mot_rr) -> Mux1/4
  Mux1/1 -> Multiport Switch/3
  [s_act_lf] -> 前轮滑转/8(s_act_lf)
  [s_opt_zhuan] -> 前轮滑转/9(s_opt_zhuan)
  后轮滑转/1(mot_lf) -> Mux2/1
  后轮滑转/3(mot_rf) -> Mux2/3
  后轮滑转/2(mot_lr) -> Mux2/2
  后轮滑转/4(mot_rr) -> Mux2/4
  后轮滑转/5(bra_pre_l1) -> Mux2/5
  后轮滑转/6(bra_pre_r1) -> Mux2/6
  Mux2/1 -> Multiport Switch/4
  [s_act_lr] -> 后轮滑转/8(s_act_lr)
  [s_opt_zhuan] -> 后轮滑转/9(s_opt_zhuan)
  Switch Case/3 -> 后轮滑转/Action
  前后轮均滑转/1(mot_lf) -> Mux3/1
  前后轮均滑转/3(mot_rf) -> Mux3/3
  前后轮均滑转/2(mot_lr) -> Mux3/2
  前后轮均滑转/4(mot_rr) -> Mux3/4
  前后轮均滑转/5(bra_pre_l1) -> Mux3/5
  前后轮均滑转/6(bra_pre_r1) -> Mux3/6
  Switch Case/4 -> 前后轮均滑转/Action
  [s_act_lf] -> 前后轮均滑转/8(s_act_lf)
  [s_act_lr] -> 前后轮均滑转/9(s_act_lr)
  [s_opt_zhuan] -> 前后轮均滑转/10(s_opt_zhuan)
  Mux3/1 -> Multiport Switch/5
  Constant4/1 -> [flag_lf]
  Constant5/1 -> [flag_lr]

== system analyze/MainControl/mode_control/backward/backward/Drive/驱动防滑控制TCS/转向TCS/左转 ==
  trq_dem_lf : Inport
  trq_dem_lr : Inport  Port=2
  trq_dem_rf : Inport  Port=3
  trq_dem_rr : Inport  Port=4
  bra_pre_l : Inport  Port=5
  bra_pre_r : Inport  Port=6
  s_act_lf : Inport  Port=7
  s_act_lr : Inport  Port=8
  s_act_rf : Inport  Port=9
  s_act_rr : Inport  Port=10
  brake_dem : Inport  Port=11
  s_opt_zhuan : Inport  Port=12
  Action Port : ActionPort  ActionType=case
  Constant{,1..3} (4 alike) : Constant  Value=s_opt_zhuan_add
  Constant4 : Constant  Value=0
  Constant5 : Constant  Value=0
  MATLAB Function : MATLAB Function  TreatAsAtomicUnit=on
  MATLAB Function1 : MATLAB Function  TreatAsAtomicUnit=on
  MATLAB Function2 : MATLAB Function  TreatAsAtomicUnit=on
  MATLAB Function3 : MATLAB Function  TreatAsAtomicUnit=on
  MATLAB Function4 : MATLAB Function  TreatAsAtomicUnit=on
  Memory{,1..3} (4 alike) : Memory  InheritSampleTime=on
  Multiport Switch : MultiPortSwitch  DataPortOrder=Zero-based contiguous  Inputs=4
  Mux{,1..3} (4 alike) : Mux  Inputs=6
  Switch Case : SwitchCase  CaseConditions={0,1,2,3}  ShowDefaultCase=off
  Terminator{,1..3} (4 alike) : Terminator
  前后轮均滑转 : Subsystem  TreatAsAtomicUnit=on
  前轮滑转 : Subsystem  TreatAsAtomicUnit=on
  后轮滑转 : Subsystem  TreatAsAtomicUnit=on
  无滑转 : Subsystem  TreatAsAtomicUnit=on
  backward_dem : Outport
  wires:
  Mux3/1 -> Multiport Switch/5
  [s_opt_zhuan] -> 前后轮均滑转/10(s_opt_zhuan)
  [s_act_rr] -> 前后轮均滑转/9(s_act_rr)
  [s_act_rf] -> 前后轮均滑转/8(s_act_rf)
  Switch Case/4 -> 前后轮均滑转/Action
  前后轮均滑转/6(bra_pre_r1) -> Mux3/6
  前后轮均滑转/5(bra_pre_l1) -> Mux3/5
  前后轮均滑转/4(mot_rr) -> Mux3/4
  前后轮均滑转/2(mot_lr) -> Mux3/2
  前后轮均滑转/3(mot_rf) -> Mux3/3
  前后轮均滑转/1(mot_lf) -> Mux3/1
  Switch Case/3 -> 后轮滑转/Action
  [s_opt_zhuan] -> 后轮滑转/9(s_opt_zhuan)
  [s_act_rr] -> 后轮滑转/8(s_act_rr)
  Mux2/1 -> Multiport Switch/4
  后轮滑转/6(bra_pre_r1) -> Mux2/6
  后轮滑转/5(bra_pre_l1) -> Mux2/5
  后轮滑转/4(mot_rr) -> Mux2/4
  后轮滑转/2(mot_lr) -> Mux2/2
  后轮滑转/3(mot_rf) -> Mux2/3
  后轮滑转/1(mot_lf) -> Mux2/1
  [s_opt_zhuan] -> 前轮滑转/9(s_opt_zhuan)
  [s_act_rf] -> 前轮滑转/8(s_act_rf)
  Mux1/1 -> Multiport Switch/3
  前轮滑转/4(mot_rr) -> Mux1/4
  前轮滑转/5(bra_pre_l1) -> Mux1/5
  前轮滑转/1(mot_lf) -> Mux1/1
  前轮滑转/2(mot_lr) -> Mux1/2
  前轮滑转/3(mot_rf) -> Mux1/3
  前轮滑转/6(bra_pre_r1) -> Mux1/6
  Switch Case/2 -> 前轮滑转/Action
  Multiport Switch/1 -> backward_dem/1
  Mux/1 -> Multiport Switch/2
  无滑转/6(bra_pre_r1) -> Mux/6
  无滑转/5(bra_pre_l1) -> Mux/5
  无滑转/3(mot_rf) -> Mux/3
  无滑转/4(mot_rr) -> Mux/4
  无滑转/2(mot_lr) -> Mux/2
  无滑转/1(mot_lf) -> Mux/1
  brake_dem/1 -> 前轮滑转/7(brake_dem), 后轮滑转/7(brake_dem), 前后轮均滑转/7(brake_dem), 无滑转/7(brake_dem)
  bra_pre_r/1 -> 前轮滑转/6(bra_pre_r), 后轮滑转/6(bra_pre_r), 前后轮均滑转/6(bra_pre_r), 无滑转/6(bra_pre_r)
  bra_pre_l/1 -> 前轮滑转/5(bra_pre_l), 后轮滑转/5(bra_pre_l), 前后轮均滑转/5(bra_pre_l), 无滑转/5(bra_pre_l)
  trq_dem_rr/1 -> 前轮滑转/4(trq_dem_rr), 后轮滑转/4(trq_dem_rr), 前后轮均滑转/4(trq_dem_rr), 无滑转/4(trq_dem_rr)
  trq_dem_rf/1 -> 前轮滑转/3(trq_dem_rf), 后轮滑转/3(trq_dem_rf), 前后轮均滑转/3(trq_dem_rf), 无滑转/3(trq_dem_rf)
  trq_dem_lr/1 -> 后轮滑转/2(trq_dem_lr), 前后轮均滑转/2(trq_dem_lr), 前轮滑转/2(trq_dem_lr), 无滑转/2(trq_dem_lr)
  trq_dem_lf/1 -> 前轮滑转/1(trq_dem_lf), 后轮滑转/1(trq_dem_lf), 前后轮均滑转/1(trq_dem_lf), 无滑转/1(trq_dem_lf)
  Switch Case/1 -> 无滑转/Action
  MATLAB Function4/1(y) -> Switch Case/1, Multiport Switch/1
  [flag_rr] -> MATLAB Function4/2(flag_rr)
  [flag_rf] -> MATLAB Function4/1(flag_rf)
  Constant3/1 -> MATLAB Function3/3(s_opt_zhuan_add)
  Memory3/1 -> MATLAB Function3/4(flag_rr_pre)
  MATLAB Function3/1(flag_rr) -> Terminator3/1, Memory3/1
  s_opt_zhuan/1 -> MATLAB Function/2(s_opt_zhuan), MATLAB Function1/2(s_opt_zhuan), MATLAB Function2/2(s_opt_zhuan), MATLAB Function3/2(s_opt_zhuan), [s_opt_zhuan]
  s_act_rr/1 -> MATLAB Function3/1(s_act_rr), [s_act_rr]
  Constant2/1 -> MATLAB Function2/3(s_opt_zhuan_add)
  Memory2/1 -> MATLAB Function2/4(flag_rf_pre)
  MATLAB Function2/1(flag_rf) -> Terminator2/1, Memory2/1
  s_act_rf/1 -> MATLAB Function2/1(s_act_rf), [s_act_rf]
  Constant1/1 -> MATLAB Function1/3(s_opt_zhuan_add)
  Memory1/1 -> MATLAB Function1/4(flag_lr_pre)
  MATLAB Function1/1(flag_lr) -> Memory1/1, Terminator1/1
  s_act_lr/1 -> MATLAB Function1/1(s_act_lr)
  Constant/1 -> MATLAB Function/3(s_opt_zhuan_add)
  Memory/1 -> MATLAB Function/4(flag_lf_pre)
  MATLAB Function/1(flag_lf) -> Memory/1, Terminator/1
  s_act_lf/1 -> MATLAB Function/1(s_act_lf)
  Constant4/1 -> [flag_rf]
  Constant5/1 -> [flag_rr]

== system analyze/MainControl/mode_control/forward/forward/Drive/驱动防滑控制TCS/直行TCS/Subsystem ==
  speed_act_lf : Inport
  v_act : Inport  Port=2
  Add : Sum
  Constant : Constant  Value=eps
  Divide : Product  Inputs=*/
  Gain : Gain  Gain=pi/30
  Gain1 : Gain  Gain=Radius
  Gain2 : Gain  Gain=1/3.6
  Subtract : Sum  Inputs=+-
  s_act_lf : Outport
  wires:
  Divide/1 -> s_act_lf/1
  Add/1 -> Divide/2
  Constant/1 -> Add/2
  Subtract/1 -> Divide/1
  Gain2/1 -> Subtract/2
  Gain1/1 -> Subtract/1, Add/1
  v_act/1 -> Gain2/1
  Gain/1 -> Gain1/1
  speed_act_lf/1 -> Gain/1

== system analyze/MainControl/mode_control/forward/forward/Drive/驱动防滑控制TCS/直行TCS/Subsystem1 ==
  speed_act_lr : Inport
  v_act : Inport  Port=2
  Add : Sum
  Constant : Constant  Value=eps
  Divide : Product  Inputs=*/
  Gain : Gain  Gain=pi/30
  Gain1 : Gain  Gain=Radius
  Gain2 : Gain  Gain=1/3.6
  Subtract : Sum  Inputs=+-
  s_act_lr : Outport
  wires:
  speed_act_lr/1 -> Gain/1
  Gain/1 -> Gain1/1
  v_act/1 -> Gain2/1
  Gain1/1 -> Add/1, Subtract/1
  Gain2/1 -> Subtract/2
  Subtract/1 -> Divide/1
  Constant/1 -> Add/2
  Add/1 -> Divide/2
  Divide/1 -> s_act_lr/1

== system analyze/MainControl/mode_control/forward/forward/Drive/驱动防滑控制TCS/直行TCS/Subsystem2 ==
  speed_act_rf : Inport
  v_act : Inport  Port=2
  Add : Sum
  Constant : Constant  Value=eps
  Divide : Product  Inputs=*/
  Gain : Gain  Gain=pi/30
  Gain1 : Gain  Gain=Radius
  Gain2 : Gain  Gain=1/3.6
  Subtract : Sum  Inputs=+-
  s_act_rf : Outport
  wires:
  Divide/1 -> s_act_rf/1
  Add/1 -> Divide/2
  Constant/1 -> Add/2
  Subtract/1 -> Divide/1
  Gain2/1 -> Subtract/2
  Gain1/1 -> Subtract/1, Add/1
  v_act/1 -> Gain2/1
  Gain/1 -> Gain1/1
  speed_act_rf/1 -> Gain/1

== system analyze/MainControl/mode_control/forward/forward/Drive/驱动防滑控制TCS/直行TCS/Subsystem3 ==
  speed_act_rr : Inport
  v_act : Inport  Port=2
  Add : Sum
  Constant : Constant  Value=eps
  Divide : Product  Inputs=*/
  Gain : Gain  Gain=pi/30
  Gain1 : Gain  Gain=Radius
  Gain2 : Gain  Gain=1/3.6
  Subtract : Sum  Inputs=+-
  s_act_rr : Outport
  wires:
  speed_act_rr/1 -> Gain/1
  Gain/1 -> Gain1/1
  v_act/1 -> Gain2/1
  Gain1/1 -> Add/1, Subtract/1
  Gain2/1 -> Subtract/2
  Subtract/1 -> Divide/1
  Constant/1 -> Add/2
  Add/1 -> Divide/2
  Divide/1 -> s_act_rr/1

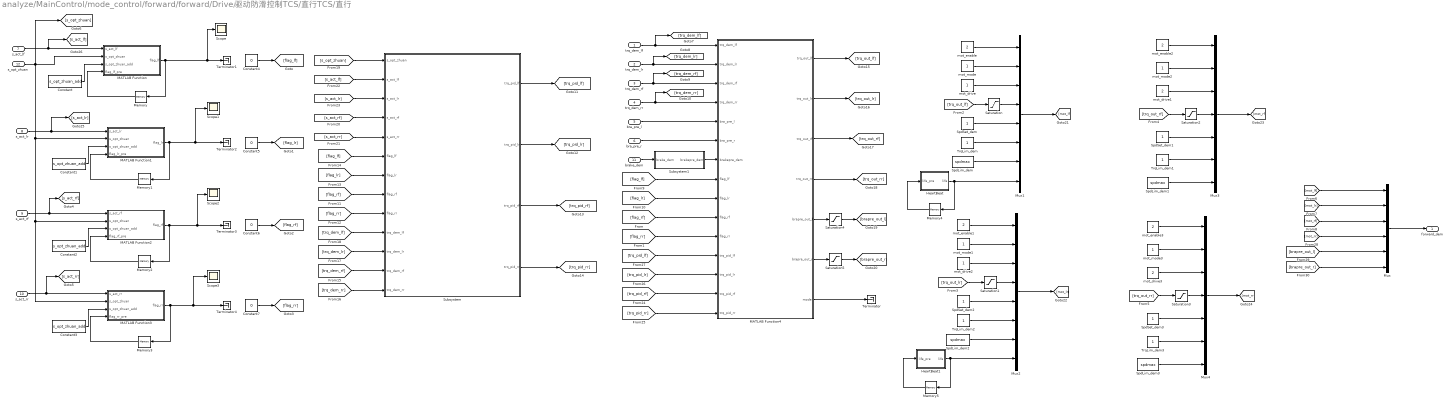
== system analyze/MainControl/mode_control/forward/forward/Drive/驱动防滑控制TCS/直行TCS/直行 ==
  trq_dem_lf : Inport
  trq_dem_lr : Inport  Port=2
  trq_dem_rf : Inport  Port=3
  trq_dem_rr : Inport  Port=4
  bra_pre_l : Inport  Port=5
  bra_pre_r : Inport  Port=6
  s_act_lf : Inport  Port=7
  s_act_lr : Inport  Port=8
  s_act_rf : Inport  Port=9
  s_act_rr : Inport  Port=10
  brake_dem : Inport  Port=11
  s_opt_zhuan : Inport  Port=12
  Constant{,1..3} (4 alike) : Constant  Value=s_opt_zhuan_add
  Constant{4..7} (4 alike) : Constant  Value=0
  HeartBeat : MATLAB Function  TreatAsAtomicUnit=on
  HeartBeat1 : MATLAB Function  TreatAsAtomicUnit=on
  MATLAB Function : MATLAB Function  TreatAsAtomicUnit=on
  MATLAB Function1 : MATLAB Function  TreatAsAtomicUnit=on
  MATLAB Function2 : MATLAB Function  TreatAsAtomicUnit=on
  MATLAB Function3 : MATLAB Function  TreatAsAtomicUnit=on
  MATLAB Function4 : MATLAB Function  TreatAsAtomicUnit=on
  Memory{,1..5} (6 alike) : Memory  InheritSampleTime=on
  Mux : Mux  Inputs=6
  Mux1 : Mux  Inputs=8
  Mux2 : Mux  Inputs=8
  Mux3 : Mux  Inputs=7
  Mux4 : Mux  Inputs=7
  Saturation{,1..3} (4 alike) : Saturate  UpperLimit=trqmax  LowerLimit=0
  Saturation4 : Saturate  UpperLimit=premax  LowerLimit=0
  Saturation5 : Saturate  UpperLimit=premax  LowerLimit=0
  Scope{,1..3} (4 alike) : Scope
      Scope settings: SaveName=ScopeData43
      Scope1 settings: SaveName=ScopeData44
      Scope2 settings: SaveName=ScopeData45
      Scope3 settings: SaveName=ScopeData46
  SpdLim_dem{,1..3} (4 alike) : Constant  Value=spdmax
  SpdSet_dem{,1..3} (4 alike) : Constant
  Subsystem : Subsystem
  Subsystem1 : Subsystem
  Terminator{,1..4} (5 alike) : Terminator
  TrqLim_dem{,1..3} (4 alike) : Constant
  mot_drive : Constant
  mot_drive1 : Constant  Value=2
  mot_drive2 : Constant
  mot_drive3 : Constant  Value=2
  mot_enable{,1..3} (4 alike) : Constant  Value=2
  mot_mode{,1..3} (4 alike) : Constant
  forward_dem : Outport
  wires:
  Mux/1 -> forward_dem/1
  [flag_rr] -> MATLAB Function4/11(flag_rr)
  [flag_rf] -> MATLAB Function4/10(flag_rf)
  Constant3/1 -> MATLAB Function3/3(s_opt_zhuan_add)
  Memory3/1 -> MATLAB Function3/4(flag_rr_pre)
  MATLAB Function3/1(flag_rr) -> Memory3/1, Terminator4/1, Scope3/1
  s_opt_zhuan/1 -> MATLAB Function/2(s_opt_zhuan), MATLAB Function1/2(s_opt_zhuan), MATLAB Function2/2(s_opt_zhuan), MATLAB Function3/2(s_opt_zhuan), [s_opt_zhuan]
  s_act_rr/1 -> MATLAB Function3/1(s_act_rr), [s_act_rr]
  Constant2/1 -> MATLAB Function2/3(s_opt_zhuan_add)
  Memory2/1 -> MATLAB Function2/4(flag_rf_pre)
  MATLAB Function2/1(flag_rf) -> Terminator3/1, Scope2/1, Memory2/1
  s_act_rf/1 -> MATLAB Function2/1(s_act_rf), [s_act_rf]
  Constant1/1 -> MATLAB Function1/3(s_opt_zhuan_add)
  Memory1/1 -> MATLAB Function1/4(flag_lr_pre)
  MATLAB Function1/1(flag_lr) -> Memory1/1, Terminator2/1, Scope1/1
  s_act_lr/1 -> [s_act_lr], MATLAB Function1/1(s_act_lr)
  Constant/1 -> MATLAB Function/3(s_opt_zhuan_add)
  Memory/1 -> MATLAB Function/4(flag_lf_pre)
  MATLAB Function/1(flag_lf) -> Terminator1/1, Scope/1, Memory/1
  s_act_lf/1 -> [s_act_lf], MATLAB Function/1(s_act_lf)
  [flag_lr] -> MATLAB Function4/9(flag_lr)
  [flag_lf] -> MATLAB Function4/8(flag_lf)
  [trq_dem_lf] -> Subsystem/10(trq_dem_lf)
  [flag_lf] -> Subsystem/6(flag_lf)
  [trq_dem_rf] -> Subsystem/12(trq_dem_rf)
  [trq_dem_lr] -> Subsystem/11(trq_dem_lr)
  [flag_lr] -> Subsystem/7(flag_lr)
  [flag_rf] -> Subsystem/8(flag_rf)
  [trq_dem_rr] -> Subsystem/13(trq_dem_rr)
  [flag_rr] -> Subsystem/9(flag_rr)
  [s_opt_zhuan] -> Subsystem/1(s_opt_zhuan)
  [s_act_rr] -> Subsystem/5(s_act_rr)
  [s_act_rf] -> Subsystem/4(s_act_rf)
  [s_act_lr] -> Subsystem/3(s_act_lr)
  [s_act_lf] -> Subsystem/2(s_act_lf)
  Subsystem/2(trq_pid_lr) -> [trq_pid_lr]
  Subsystem/1(trq_pid_lf) -> [trq_pid_lf]
  Subsystem/4(trq_pid_rr) -> [trq_pid_rr]
  Subsystem/3(trq_pid_rf) -> [trq_pid_rf]
  [trq_pid_lf] -> MATLAB Function4/12(trq_pid_lf)
  [trq_pid_lr] -> MATLAB Function4/13(trq_pid_lr)
  [trq_pid_rf] -> MATLAB Function4/14(trq_pid_rf)
  [trq_pid_rr] -> MATLAB Function4/15(trq_pid_rr)
  trq_dem_lf/1 -> MATLAB Function4/1(trq_dem_lf), [trq_dem_lf]
  trq_dem_lr/1 -> MATLAB Function4/2(trq_dem_lr), [trq_dem_lr]
  trq_dem_rf/1 -> MATLAB Function4/3(trq_dem_rf), [trq_dem_rf]
  trq_dem_rr/1 -> MATLAB Function4/4(trq_dem_rr), [trq_dem_rr]
  bra_pre_l/1 -> MATLAB Function4/5(bra_pre_l)
  bra_pre_r/1 -> MATLAB Function4/6(bra_pre_r)
  SpdLim_dem3/1 -> Mux4/7
  TrqLim_dem3/1 -> Mux4/6
  Mux4/1 -> [mot_rr]
  SpdSet_dem3/1 -> Mux4/5
  mot_enable3/1 -> Mux4/1
  [trq_out_rr] -> Saturation3/1
  mot_mode3/1 -> Mux4/2
  mot_drive3/1 -> Mux4/3
  SpdLim_dem2/1 -> Mux2/7
  Memory5/1 -> HeartBeat1/1(life_pre)
  HeartBeat1/1(life) -> Memory5/1, Mux2/8
  TrqLim_dem2/1 -> Mux2/6
  Mux2/1 -> [mot_lr]
  SpdSet_dem2/1 -> Mux2/5
  mot_enable1/1 -> Mux2/1
  [trq_out_lr] -> Saturation1/1
  mot_mode1/1 -> Mux2/2
  mot_drive2/1 -> Mux2/3
  SpdLim_dem1/1 -> Mux3/7
  TrqLim_dem1/1 -> Mux3/6
  Mux3/1 -> [mot_rf]
  SpdSet_dem1/1 -> Mux3/5
  mot_enable2/1 -> Mux3/1
  [trq_out_rf] -> Saturation2/1
  mot_mode2/1 -> Mux3/2
  mot_drive1/1 -> Mux3/3
  SpdLim_dem/1 -> Mux1/7
  Memory4/1 -> HeartBeat/1(life_pre)
  HeartBeat/1(life) -> Memory4/1, Mux1/8
  TrqLim_dem/1 -> Mux1/6
  Mux1/1 -> [mot_lf]
  SpdSet_dem/1 -> Mux1/5
  mot_enable/1 -> Mux1/1
  [trq_out_lf] -> Saturation/1
  mot_mode/1 -> Mux1/2
  mot_drive/1 -> Mux1/3
  MATLAB Function4/1(trq_out_lf) -> [trq_out_lf]
  MATLAB Function4/2(trq_out_lr) -> [trq_out_lr]
  MATLAB Function4/3(trq_out_rf) -> [trq_out_rf]
  MATLAB Function4/4(trq_out_rr) -> [trq_out_rr]
  MATLAB Function4/5(brapre_out_l) -> Saturation4/1
  MATLAB Function4/6(brapre_out_r) -> Saturation5/1
  [mot_lf] -> Mux/1
  [mot_lr] -> Mux/2
  [mot_rf] -> Mux/3
  [mot_rr] -> Mux/4
  [brapre_out_l] -> Mux/5
  [brapre_out_r] -> Mux/6
  Subsystem1/1(brakepre_dem) -> MATLAB Function4/7(brakepre_dem)
  brake_dem/1 -> Subsystem1/1(brake_dem)
  MATLAB Function4/7(mode) -> Terminator/1
  Saturation/1 -> Mux1/4
  Saturation2/1 -> Mux3/4
  Saturation1/1 -> Mux2/4
  Saturation3/1 -> Mux4/4
  Saturation4/1 -> [brapre_out_l]
  Saturation5/1 -> [brapre_out_r]
  Constant4/1 -> [flag_lf]
  Constant5/1 -> [flag_lr]
  Constant6/1 -> [flag_rf]
  Constant7/1 -> [flag_rr]

== system analyze/MainControl/mode_control/forward/forward/Drive/驱动防滑控制TCS/转向TCS/Subsystem ==
  speed_act_lf : Inport
  v_act : Inport  Port=2
  Add : Sum
  Constant : Constant  Value=eps
  Divide : Product  Inputs=*/
  Gain : Gain  Gain=pi/30
  Gain1 : Gain  Gain=Radius
  Gain2 : Gain  Gain=1/3.6
  Subtract : Sum  Inputs=+-
  s_act_lf : Outport
  wires:
  speed_act_lf/1 -> Gain/1
  Gain/1 -> Gain1/1
  v_act/1 -> Gain2/1
  Gain1/1 -> Add/1, Subtract/1
  Gain2/1 -> Subtract/2
  Subtract/1 -> Divide/1
  Constant/1 -> Add/2
  Add/1 -> Divide/2
  Divide/1 -> s_act_lf/1

== system analyze/MainControl/mode_control/forward/forward/Drive/驱动防滑控制TCS/转向TCS/Subsystem1 ==
  speed_act_lr : Inport
  v_act : Inport  Port=2
  Add : Sum
  Constant : Constant  Value=eps
  Divide : Product  Inputs=*/
  Gain : Gain  Gain=pi/30
  Gain1 : Gain  Gain=Radius
  Gain2 : Gain  Gain=1/3.6
  Subtract : Sum  Inputs=+-
  s_act_lr : Outport
  wires:
  Divide/1 -> s_act_lr/1
  Add/1 -> Divide/2
  Constant/1 -> Add/2
  Subtract/1 -> Divide/1
  Gain2/1 -> Subtract/2
  Gain1/1 -> Subtract/1, Add/1
  v_act/1 -> Gain2/1
  Gain/1 -> Gain1/1
  speed_act_lr/1 -> Gain/1

== system analyze/MainControl/mode_control/forward/forward/Drive/驱动防滑控制TCS/转向TCS/Subsystem2 ==
  speed_act_rf : Inport
  v_act : Inport  Port=2
  Add : Sum
  Constant : Constant  Value=eps
  Divide : Product  Inputs=*/
  Gain : Gain  Gain=pi/30
  Gain1 : Gain  Gain=Radius
  Gain2 : Gain  Gain=1/3.6
  Subtract : Sum  Inputs=+-
  s_act_rf : Outport
  wires:
  speed_act_rf/1 -> Gain/1
  Gain/1 -> Gain1/1
  v_act/1 -> Gain2/1
  Gain1/1 -> Add/1, Subtract/1
  Gain2/1 -> Subtract/2
  Subtract/1 -> Divide/1
  Constant/1 -> Add/2
  Add/1 -> Divide/2
  Divide/1 -> s_act_rf/1

== system analyze/MainControl/mode_control/forward/forward/Drive/驱动防滑控制TCS/转向TCS/Subsystem3 ==
  speed_act_rr : Inport
  v_act : Inport  Port=2
  Add : Sum
  Constant : Constant  Value=eps
  Divide : Product  Inputs=*/
  Gain : Gain  Gain=pi/30
  Gain1 : Gain  Gain=Radius
  Gain2 : Gain  Gain=1/3.6
  Subtract : Sum  Inputs=+-
  s_act_rr : Outport
  wires:
  Divide/1 -> s_act_rr/1
  Add/1 -> Divide/2
  Constant/1 -> Add/2
  Subtract/1 -> Divide/1
  Gain2/1 -> Subtract/2
  Gain1/1 -> Subtract/1, Add/1
  v_act/1 -> Gain2/1
  Gain/1 -> Gain1/1
  speed_act_rr/1 -> Gain/1
